simulink model "Vjezba5"  (R2016b)
settings: Solver=FixedStepAuto  StartTime=0.0  StopTime=100  FixedStep=0.0001  RelTol=1e-3
libraries: simulink_extras x3, simulink x3
settings Model: Creator=Luka  LastModifiedBy=Luka

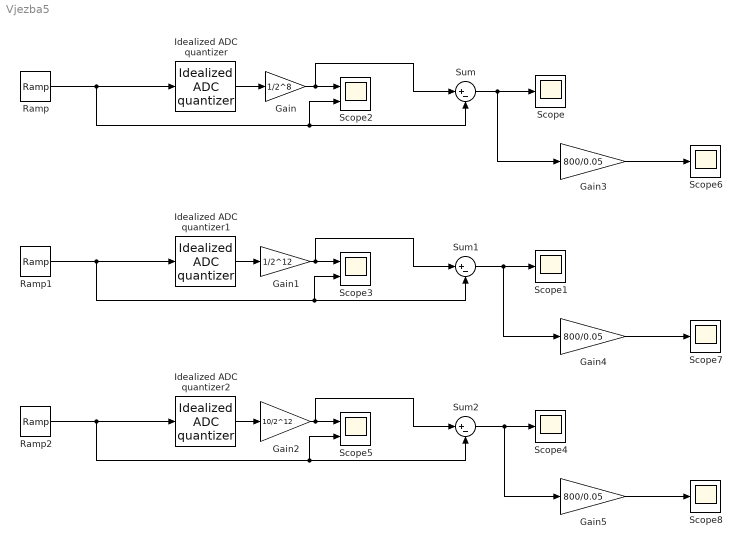
== system Vjezba5 ==
  Gain : Gain  Gain=1/2^8
  Gain1 : Gain  Gain=1/2^12
  Gain2 : Gain  Gain=10/2^12
  Gain3 : Gain  Gain=800/0.05
  Gain4 : Gain  Gain=800/0.05
  Gain5 : Gain  Gain=800/0.05
  Idealized ADC quantizer : simulink_extras/Additional Discrete/Idealized ADC quantizer  NumberOfConverterBits=8  Vmin=0  Vmax=1  OutputDataType=int16  OutputNegativeValues=off
  Idealized ADC quantizer1 : simulink_extras/Additional Discrete/Idealized ADC quantizer  NumberOfConverterBits=12  Vmin=0  Vmax=1  OutputDataType=int16  OutputNegativeValues=off
  Idealized ADC quantizer2 : simulink_extras/Additional Discrete/Idealized ADC quantizer  NumberOfConverterBits=12  Vmin=0  Vmax=10  OutputDataType=int16  OutputNegativeValues=off
  Ramp : simulink/Sources/Ramp  slope=0.05/800  start=0  X0=0
  Ramp1 : simulink/Sources/Ramp  slope=0.05/800  start=0  X0=0
  Ramp2 : simulink/Sources/Ramp  slope=0.05/800  start=0  X0=0
  Scope{,1,4,6..8} (6 alike) : Scope
  Scope2 : Scope  NumInputPorts=2
  Scope3 : Scope  NumInputPorts=2
  Scope5 : Scope  NumInputPorts=2
  Sum : Sum  Inputs=|+-
  Sum1 : Sum  Inputs=|+-
  Sum2 : Sum  Inputs=|+-
  wires:
  Ramp/1 -> Sum/2, Scope2/2, Idealized ADC quantizer/1
  Idealized ADC quantizer/1 -> Gain/1
  Gain/1 -> Sum/1, Scope2/1
  Sum/1 -> Gain3/1, Scope/1
  Gain1/1 -> Scope3/1, Sum1/1
  Idealized ADC quantizer1/1 -> Gain1/1
  Ramp1/1 -> Idealized ADC quantizer1/1, Scope3/2, Sum1/2
  Ramp2/1 -> Sum2/2, Scope5/2, Idealized ADC quantizer2/1
  Idealized ADC quantizer2/1 -> Gain2/1
  Gain2/1 -> Sum2/1, Scope5/1
  Gain3/1 -> Scope6/1
  Gain4/1 -> Scope7/1
  Sum1/1 -> Gain4/1, Scope1/1
  Sum2/1 -> Gain5/1, Scope4/1
  Gain5/1 -> Scope8/1
